simulink model "Aufschw_2021b"  (R2021b)
settings: Solver=FixedStepAuto  StartTime=0.0  StopTime=5  FixedStep=1/1e4  RelTol=1e-3
model workspace (MATLAB code in the model file):
  | global Theta_1;
  | Theta_1=pi;
undefined symbols (not defined in the file): A, B, C, E0, k, L, Phi, Phi_Punkt, start_deg, Theta, Theta_Punkt, V_m, x_c
libraries: embmathops x3
settings Model: Creator=basti  LastModifiedBy=cyril

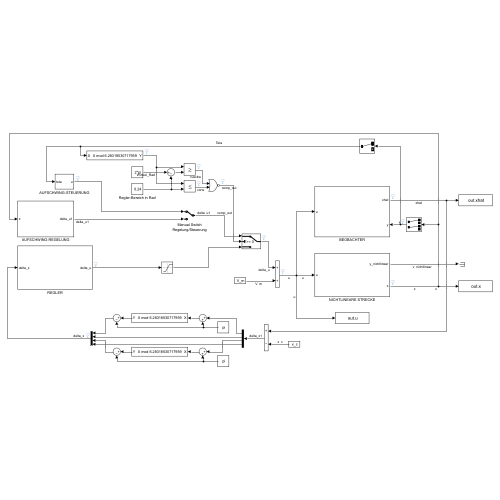
[thumbnail: Simulink's stored preview of the top-level diagram]
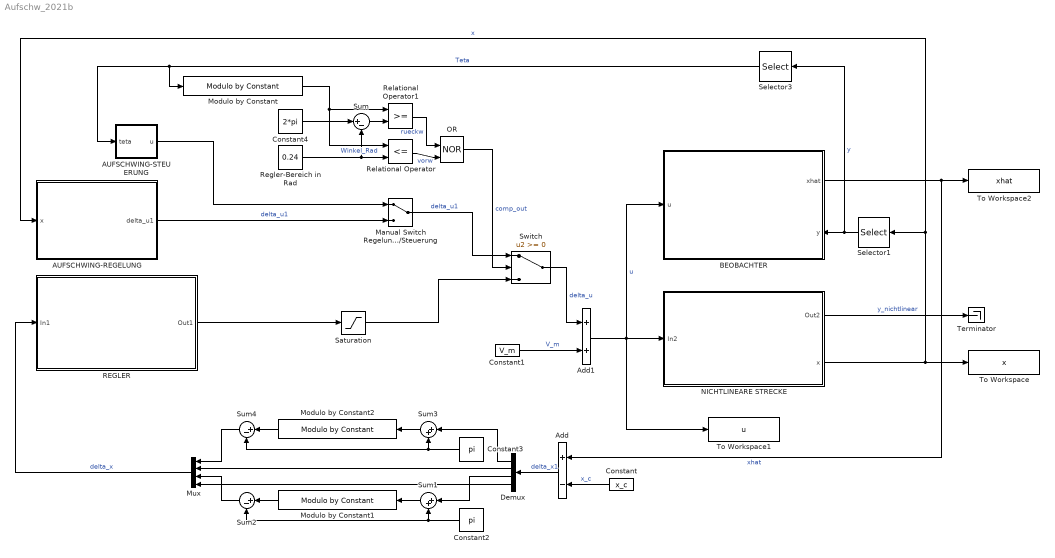
== system Aufschw_2021b ==
  AUFSCHWING-REGELUNG : Subsystem
  AUFSCHWING-STEUERUNG : Subsystem
  Add : Sum  Inputs=+-
  Add1 : Sum
  BEOBACHTER : Subsystem
      settings: PortSchema="{\"entries\":[{\"content\":{\"sides\":[{\"content\":{\"connectorIds\":[\"Out1\",\"In1\"]},\"type\":\"ConnectorPlacement.EquallySpacedRectSide\",\"uuid\":\"bf04db51-b94f-4a7f-8932-7ebd32ee2318\"},{\"content\":{\"connectorIds\":[\"In2\"],\"side\":\"RIGHT\"},\"type\":\"ConnectorPlacement.EquallySpacedRectSide\",\"uuid\":\"77aa8635-bee0-48fe-bbc1-b57ac7cbc0f7\"},{\"content\":{\"connectorIds\":[],\"side\":\"TOP\"},\"type\":\"ConnectorPlacement.EquallySpacedRectSide\",\"uuid\":\"d421fec2-fc4e-412a-a9ec-fddb198b3152\"}]},\"type\":\"ConnectorPlacement.EquallySpacedConnector\",\"uuid\":\"8f05bc36-bea1-4787-80e3-58e983489b6b\"}],\"packageUris\":[\"http://schema.mathworks.com/mf0/Connector/R2020b\"],\"version\":\"1.0\"}"
  Constant : Constant  Value=x_c
  Constant1 : Constant  Value=V_m
  Constant2 : Constant  Value=pi
  Constant3 : Constant  Value=pi
  Constant4 : Constant  Value=2*pi
  Demux : Demux
  Manual Switch Regelung/Steuerung : ManualSwitch
  Modulo by Constant : embmathops/Modulo by Constant  Denominator=2*pi  SimulateUsing=Code generation
      settings: SourceProductBaseCode=SL
  Modulo by Constant1 : embmathops/Modulo by Constant  Denominator=2*pi  SimulateUsing=Code generation
      settings: SourceProductBaseCode=SL
  Modulo by Constant2 : embmathops/Modulo by Constant  Denominator=2*pi  SimulateUsing=Code generation
      settings: SourceProductBaseCode=SL
  Mux : Mux
  NICHTLINEARE STRECKE : Subsystem
  OR : Logic  Operator=NOR  IconShape=distinctive  AllPortsSameDT=off  OutDataTypeStr=boolean
  REGLER : Subsystem
  Regler-Bereich in Rad : Constant  Value=0.24
  Relational Operator : RelationalOperator  Operator=<=  OutDataTypeStr=boolean  RndMeth=Simplest
  Relational Operator1 : RelationalOperator  OutDataTypeStr=boolean  RndMeth=Simplest
  Saturation : Saturate  UpperLimit=40  LowerLimit=-40  LinearizeAsGain=off
  Selector1 : Selector  InputPortWidth=4  IndexOptions=Index vector (dialog)  Indices=[1 3]  OutputSizes=1
  Selector3 : Selector  InputPortWidth=2  IndexOptions=Index vector (dialog)  Indices=1  OutputSizes=1
  Sum : Sum  Inputs=|+-
  Sum1 : Sum  Inputs=|++
  Sum2 : Sum  Inputs=|+-
  Sum3 : Sum  Inputs=|++
  Sum4 : Sum  Inputs=|+-
  Switch : Switch
  Terminator : Terminator
  To Workspace : ToWorkspace  VariableName=x  SaveFormat=Timeseries  SampleTime=-1
  To Workspace1 : ToWorkspace  VariableName=u  SaveFormat=Timeseries  SampleTime=-1
  To Workspace2 : ToWorkspace  VariableName=xhat  SaveFormat=Timeseries  SampleTime=-1
  wires:
  NICHTLINEARE STRECKE/1(Out2) -> Terminator/1  "y_nichtlinear"
  Constant/1 -> Add/2  "x_c"
  NICHTLINEARE STRECKE/2(x) -> AUFSCHWING-REGELUNG/1(x), Selector1/1, To Workspace/1  "x"
  Mux/1 -> REGLER/1(In1)  "delta_x"
  Add1/1 -> BEOBACHTER/2(u), To Workspace1/1, NICHTLINEARE STRECKE/1(In2)  "u"
  Constant1/1 -> Add1/2  "V_m"
  Switch/1 -> Add1/1  "delta_u"
  Manual Switch Regelung/Steuerung/1 -> Switch/1  "delta_u1"
  REGLER/1(Out1) -> Saturation/1
  Demux/1 -> Sum3/1
  OR/1 -> Switch/2  "comp_out"
  Regler-Bereich in Rad/1 -> Relational Operator/2, Sum/2
  Modulo by Constant/1 -> Relational Operator/1, Relational Operator1/1  "Winkel_Rad"
  Relational Operator1/1 -> OR/1  "rueckw"
  Relational Operator/1 -> OR/2  "vorw"
  Sum/1 -> Relational Operator1/2
  Constant4/1 -> Sum/1
  Saturation/1 -> Switch/3
  Demux/2 -> Mux/2
  Add/1 -> Demux/1  "delta_x1"
  Sum1/1 -> Modulo by Constant1/1
  Modulo by Constant1/1 -> Sum2/1
  Constant2/1 -> Sum2/2, Sum1/2
  Sum3/1 -> Modulo by Constant2/1
  Modulo by Constant2/1 -> Sum4/1
  Constant3/1 -> Sum4/2, Sum3/2
  Sum4/1 -> Mux/1
  Demux/3 -> Sum1/1
  Sum2/1 -> Mux/3
  Demux/4 -> Mux/4
  Selector1/1 -> Selector3/1, BEOBACHTER/1(y)  "y"
  BEOBACHTER/1(xhat) -> Add/1, To Workspace2/1  "xhat"
  AUFSCHWING-STEUERUNG/1(u) -> Manual Switch Regelung/Steuerung/1
  AUFSCHWING-REGELUNG/1(delta_u1) -> Manual Switch Regelung/Steuerung/2  "delta_u1"
  Selector3/1 -> Modulo by Constant/1, AUFSCHWING-STEUERUNG/1(teta)  "Teta"

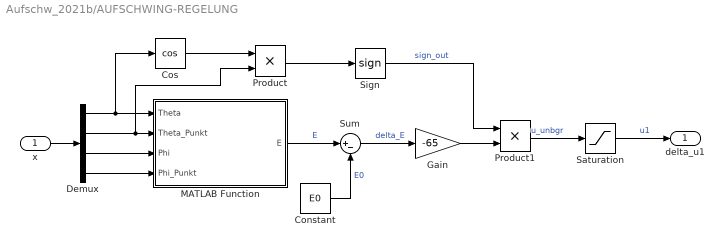
== system Aufschw_2021b/AUFSCHWING-REGELUNG ==
  x : Inport
  Constant : Constant  Value=E0
  Cos : Trigonometry  Operator=cos
  Demux : Demux
  Gain : Gain  Gain=-65
  MATLAB Function : MATLAB Function  TreatAsAtomicUnit=on
  Product : Product
  Product1 : Product
  Saturation : Saturate  UpperLimit=50  LowerLimit=-50  LinearizeAsGain=off
  Sign : Signum
  Sum : Sum  Inputs=|+-
  delta_u1 : Outport
  wires:
  x/1 -> Demux/1
  Demux/1 -> Cos/1, MATLAB Function/1(Theta)
  Demux/3 -> MATLAB Function/3(Phi)
  Demux/4 -> MATLAB Function/4(Phi_Punkt)
  MATLAB Function/1(E) -> Sum/1  "E"
  Sum/1 -> Gain/1  "delta_E"
  Constant/1 -> Sum/2  "E0"
  Sign/1 -> Product1/1  "sign_out"
  Gain/1 -> Product1/2
  Product1/1 -> Saturation/1  "u_unbgr"
  Saturation/1 -> delta_u1/1  "u1"
  Cos/1 -> Product/1
  Product/1 -> Sign/1
  Demux/2 -> Product/2, MATLAB Function/2(Theta_Punkt)

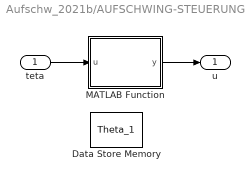
== system Aufschw_2021b/AUFSCHWING-STEUERUNG ==
  teta : Inport  OutDataTypeStr=double  PortDimensions=1
  Data Store Memory : DataStoreMemory  DataStoreName=Theta_1  WriteAfterWriteMsg=warning  InitialValue=pi  ShowAdditionalParam=off  OutDataTypeStr=double  Dimensions=1
  MATLAB Function : MATLAB Function  TreatAsAtomicUnit=on
  u : Outport
  wires:
  teta/1 -> MATLAB Function/1(u)
  MATLAB Function/1(y) -> u/1

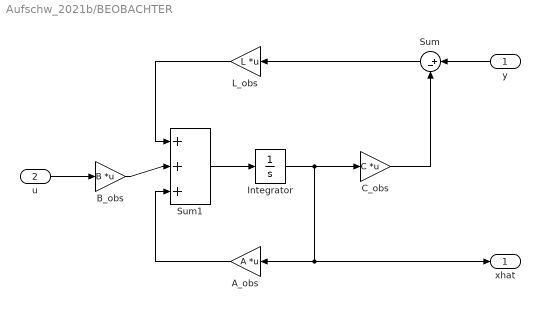
== system Aufschw_2021b/BEOBACHTER ==
  y : Inport
  u : Inport  Port=2
  A_obs : Gain  Gain=A  Multiplication=Matrix(K*u)
  B_obs : Gain  Gain=B  Multiplication=Matrix(K*u)
  C_obs : Gain  Gain=C  Multiplication=Matrix(K*u)
  Integrator : Integrator
  L_obs : Gain  Gain=L  Multiplication=Matrix(K*u)
  Sum : Sum  Inputs=|+-
  Sum1 : Sum  Inputs=|+++
  xhat : Outport
  wires:
  y/1 -> Sum/1
  C_obs/1 -> Sum/2
  Integrator/1 -> xhat/1, A_obs/1, C_obs/1
  B_obs/1 -> Sum1/2
  A_obs/1 -> Sum1/3
  Sum/1 -> L_obs/1
  L_obs/1 -> Sum1/1
  u/1 -> B_obs/1
  Sum1/1 -> Integrator/1

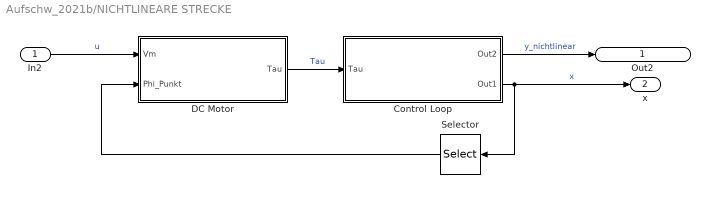
== system Aufschw_2021b/NICHTLINEARE STRECKE ==
  In2 : Inport
  Control Loop : Subsystem
  DC Motor : Subsystem
  Selector : Selector  InputPortWidth=4  IndexOptions=Index vector (dialog)  Indices=4  OutputSizes=1
  Out2 : Outport
  x : Outport  Port=2
  wires:
  In2/1 -> DC Motor/1(Vm)  "u"
  DC Motor/1(Tau) -> Control Loop/1(Tau)  "Tau"
  Control Loop/2(Out1) -> x/1, Selector/1  "x"
  Selector/1 -> DC Motor/2(Phi_Punkt)
  Control Loop/1(Out2) -> Out2/1  "y_nichtlinear"

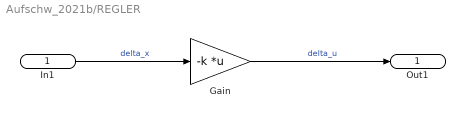
== system Aufschw_2021b/REGLER ==
  In1 : Inport
  Gain : Gain  Gain=-k  Multiplication=Matrix(K*u) (u vector)
  Out1 : Outport
  wires:
  Gain/1 -> Out1/1  "delta_u"
  In1/1 -> Gain/1  "delta_x"

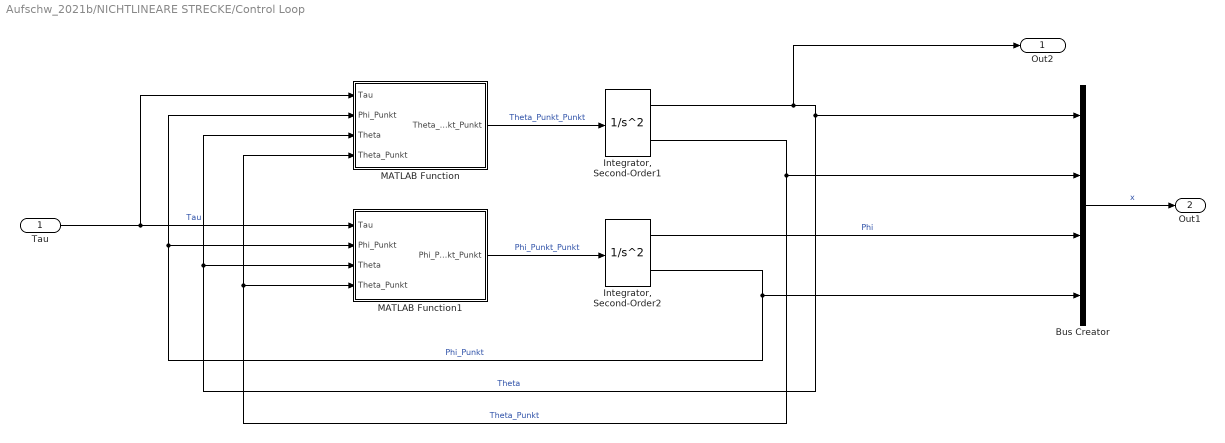
== system Aufschw_2021b/NICHTLINEARE STRECKE/Control Loop ==
  Tau : Inport
  Bus Creator : BusCreator  Inputs=Theta,Theta_Punkt,Phi,Phi_Punkt
  "Integrator, Second-Order1" : SecondOrderIntegrator  ICX=x_c(1)+(start_deg*pi/180)  ICDXDT=x_c(2)
  "Integrator, Second-Order2" : SecondOrderIntegrator  ICX=x_c(3)  ICDXDT=x_c(4)
  MATLAB Function : MATLAB Function  TreatAsAtomicUnit=on
  MATLAB Function1 : MATLAB Function  TreatAsAtomicUnit=on
  Out2 : Outport
  Out1 : Outport  Port=2
  wires:
  MATLAB Function/1(Theta_Punkt_Punkt) -> "Integrator, Second-Order1"/1  "Theta_Punkt_Punkt"
  MATLAB Function1/1(Phi_Punkt_Punkt) -> "Integrator, Second-Order2"/1  "Phi_Punkt_Punkt"
  "Integrator, Second-Order2"/2 -> MATLAB Function1/2(Phi_Punkt), MATLAB Function/2(Phi_Punkt), Bus Creator/4  "Phi_Punkt"
  "Integrator, Second-Order1"/2 -> MATLAB Function/4(Theta_Punkt), MATLAB Function1/4(Theta_Punkt), Bus Creator/2  "Theta_Punkt"
  Tau/1 -> MATLAB Function/1(Tau), MATLAB Function1/1(Tau)  "Tau"
  Bus Creator/1 -> Out1/1  "x"
  "Integrator, Second-Order1"/1 -> Out2/1, Bus Creator/1, MATLAB Function1/3(Theta), MATLAB Function/3(Theta)  "Theta"
  "Integrator, Second-Order2"/1 -> Bus Creator/3  "Phi"

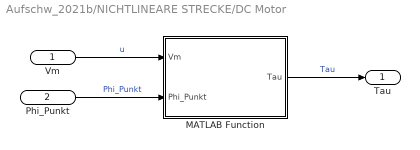
== system Aufschw_2021b/NICHTLINEARE STRECKE/DC Motor ==
  Vm : Inport
  Phi_Punkt : Inport  Port=2
  MATLAB Function : MATLAB Function  TreatAsAtomicUnit=on
  Tau : Outport
  wires:
  Vm/1 -> MATLAB Function/1(Vm)  "u"
  Phi_Punkt/1 -> MATLAB Function/2(Phi_Punkt)  "Phi_Punkt"
  MATLAB Function/1(Tau) -> Tau/1  "Tau"

== matlab function Aufschw_2021b/NICHTLINEARE STRECKE/Control Loop/MATLAB Function1 ==
  data: Tau input; Phi_Punkt_Punkt output; Phi_Punkt input; Theta input; Theta_Punkt input
function Phi_Punkt_Punkt = fcn(Tau, Phi_Punkt, Theta, Theta_Punkt)
    % Konstanten aufrufen
    c = Konstanten();
    
    % Berechnung
    Phi_Punkt_Punkt = (((c.m1*c.l1+c.m2*c.l2)*c.g*sin(Theta)-c.c1*Theta_Punkt-(c.m1*c.l1^2+c.m2*c.l2^2+c.J1+c.J2)*(Tau-c.c2*Phi_Punkt)/c.J2)/c.J2)/(1-(c.m1*c.l1^2+c.m2*c.l2^2+c.J1+c.J2)/c.J2);

== matlab function Aufschw_2021b/NICHTLINEARE STRECKE/Control Loop/MATLAB Function ==
  data: Tau input; Theta_Punkt_Punkt output; Phi_Punkt input; Theta input; Theta_Punkt input
function Theta_Punkt_Punkt = fcn(Tau, Phi_Punkt, Theta, Theta_Punkt)
    % Konstanten aufrufen
    c = Konstanten();
    
    % Berechnung
    Theta_Punkt_Punkt = ((Tau-c.c2*Phi_Punkt-(c.m1*c.l1+c.m2*c.l2)*c.g*sin(Theta)+c.c1*Theta_Punkt)/c.J2)/(1-(c.m1*c.l1^2+c.m2*c.l2^2+c.J1+c.J2)/c.J2);

== matlab function Aufschw_2021b/NICHTLINEARE STRECKE/DC Motor/MATLAB Function ==
  data: Vm input; Tau output; Phi_Punkt input
function Tau = fcn(Vm, Phi_Punkt)
    % Konstanten
    c = Konstanten();
    
    % Berechnung
    Tau = c.Kt*(Vm-c.Kb*Phi_Punkt)/c.Ra;

== matlab function Aufschw_2021b/AUFSCHWING-REGELUNG/MATLAB Function ==
  data: Theta input; Theta_Punkt input; Phi input; E output; Phi_Punkt input
function E = fcn(Theta, Theta_Punkt, Phi, Phi_Punkt)
    % Konstanten aufrufen
    c = Konstanten();
    
    % Berechnung

    T1=(c.m1/2)*(c.l1*Theta_Punkt)^2+(c.m2/2)*(c.l2*Theta_Punkt)^2;
    V=(c.m1*c.l1+c.m2*c.l2)*c.g*cos(Theta);
    E=T1+V;

== matlab function Aufschw_2021b/AUFSCHWING-STEUERUNG/MATLAB Function ==
  settings: updateMethod=DISCRETE
  data: u input; y output; Theta_1 data_store_memory
function y = fcn(u)

global Theta_1;

if (u>Theta_1)
    y=-40;
else
    y=40;
end
Theta_1=u;
